simulink library "mpc555toucan"  (Simulink 6.0)
settings: Solver=ode45  SolverMode=SingleTasking  StartTime=0.0  StopTime=10.0  RelTol=1e-3
libraries: passthrough x20, driver_interface_library x10, canblocks x3, mpc555toucan x3, canblocks_extras x2, mpc555extras x2, mpc555interrupts x1, simulink x1, config_library x1
settings Model: Creator=The MathWorks Inc.  LastModifiedBy=batserve  ExtModeAutoUpdateStatusClock=off  ProdHWDeviceType=Specified
settings OptimizationCC: BooleanDataType=off
settings DebuggingCC: CheckExecutionContextPreStartOutputMsg=on  CheckExecutionContextRuntimeOutputMsg=on  SolverPrmCheckMsg=none
settings HardwareCC: ProdHWDeviceType=Specified  TargetUnknown=on

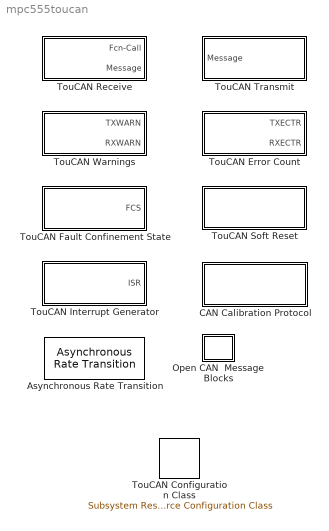
== system mpc555toucan ==
  Asynchronous Rate Transition : mpc555interrupts/Asynchronous Rate Transition  sample_time=-1
  CAN Calibration Protocol : Subsystem  TreatAsAtomicUnit=on  PropExecContextAcrossSSBoundary=on  mask(CAN Calibration Protocol (MPC555)){CCP_STATION_ID=hex2dec('1'), module=A, ccp_cro_id=hex2dec('6FA'), ccp_cro_message_type=Extended (29-bit identifier), ccp_return_id=hex2dec('6FB'), ccp_return_message_type=Extended (29-bit identifier), TOTAL_NUM_ODTS=8, cro_sample_time=0.01}
      mask prompts: CCP_STATION_ID "CCP station address (16-bit integer):"; module "TouCAN module:"; ccp_cro_id "CAN message identifier (CRO):"; ccp_cro_message_type "CAN message type (CRO):"; ccp_return_id "CAN message identifier (DTO/DAQ):"; ccp_return_message_type "CAN message type (DTO/DAQ):"; TOTAL_NUM_ODTS "Total Number of Object Descriptor Tables (ODTs):"; cro_sample_time "CRO sample time:"
      mask help:
      | Implements CAN Calibration Protocol (CCP v2.1) on the target processor.
      |
      | This block processes Command Receive Object (CRO) messages and outputs the resulting Data Transmission Object (DTO) and Data Acquisition (DAQ) messages.
      mask init:
      | % Propagate DAQ / DTO message type to underlying blocks
      | set_param([gcb, '/DAQ Processing/Send DAQ Message/CAN Message Packing'], 'message_type', ccp_return_message_type);
      | set_param([gcb, '/DTO Processing/CCP (Termination)/CAN Transmit/DTO_Constructor'], 'message_type', ccp_return_message_type);
      | % Propagate CRO message type to underlying blocks
      | set_param([gcb, '/TouCAN Receive'], 'message_type', ccp_cro_message_type);
      | % Propagate TouCAN module to underlying blocks
      | set_param([gcb, '/DAQ Processing/Send DAQ Message/TouCAN Transmit'], 'module', module);
      | set_param([gcb, '/DTO Processing/CCP (Termination)/CAN Transmit/TouCAN Transmit'], 'module', module);
      | set_param([gcb, '/TouCAN Receive'], 'module', module);
      | 
      | % check for a Resource Config block, and make sure it is MPC555
      | target = RTWConfigurationCB('get_target', gcb);
      | target.checkName('MPC555');
      | 
      | ccp_mpc555_init_mask('check_prog_prep_bit_timing', gcb, target);
      settings: CopyFcn=ccp_init_mask('copyfcn', gcb)
      mask Help: helpview([docroot '/toolbox/mpc555dk/mpc555dk.map'], 'target_CCP');
      mask StyleString: edit,popup(A|B|C),edit,popup(Standard (11-bit identifier)|Extended (29-bit identifier)),edit,popup(Standard (11-bit identifier)|Extended (29-bit identifier)),edit,edit
      mask Display: disp('CCP');
  Open CAN  Message Blocks : Subsystem  PropExecContextAcrossSSBoundary=on
      mask init:
      | [x colormap] = imread([matlabroot '\toolbox\rtw\targets\common\tgtcommon\model.gif']);
      | rgb = ind2rgb(x, colormap);
      settings: OpenFcn=canblocks
      mask Display: image(rgb)
  TouCAN Configuration Class : config_library/Subsystem Resource Configuration Class  Tag=CONFIGURATION DATA CLASS  dClassName=MPC555dkConfig.TOUCAN  rClassName=MPC555dkConfig.TOUCAN_RESOURCES
  TouCAN Error Count : Subsystem  PropExecContextAcrossSSBoundary=on  mask(MPC555 TouCAN Error Count (Transmit/Receive)){module=A, t=0.1, enablePassThru=off}
      mask prompts: t "Sample time:"; enablePassThru "Enable pass through (show simulation input)"
      mask help: Read the transmit/receive error counter registers (TXECTR/RXECTR) on the selected TouCAN module.
      mask init:
      | simulinkPortControl(gcbh,'enable','PassThroughRXECTR',enablePassThru);
      | simulinkPortControl(gcbh,'enable','PassThroughTXECTR',enablePassThru);
      | 
      | dispstr = sprintf('TouCAN_%s\nError Count', module);
      | 
      | if (enablePassThru)
      | 	passThroughDeprecationWarning;
      | end;
      | 
      | % check for a Resource Config block, and make sure it is MPC555
      | target = RTWConfigurationCB('get_target', gcb);
      | target.checkName('MPC555');
      | 
      | % Verify the modules selection is correct
      | mpc5xx_2can_verify_modules(gcb);
      mask Help: helpview([docroot '/toolbox/mpc555dk/mpc555dk.map'], 'TouCAN_Err_Ctr');
      mask StyleString: popup(A|B|C),edit,checkbox
      mask Display:
      | disp(dispstr)
      | port_label('output',1,'Tx');
      | port_label('output',2,'Rx');
  TouCAN Fault Confinement State : Subsystem  PropExecContextAcrossSSBoundary=on  mask(MPC555 TouCAN Fault Confinement State){module=A, t=0.1, enablePassThru=off}
      mask prompts: t "Sample time:"; enablePassThru "Enable pass through (show simulation input)"
      mask help: Indicates the fault confinement state of a TouCAN module.
      mask init:
      | simulinkPortControl(gcbh,'enable','PassThrough',enablePassThru);
      | 
      | dispstr = sprintf('TouCAN_%s\nFault \nConfinement State', module);
      | 
      | if (enablePassThru)
      | 	passThroughDeprecationWarning;
      | end;
      | 
      | % check for a Resource Config block, and make sure it is MPC555
      | target = RTWConfigurationCB('get_target', gcb);
      | target.checkName('MPC555');
      | 
      | % Verify the modules selection is correct
      | mpc5xx_2can_verify_modules(gcb);
      mask Help: helpview([docroot '/toolbox/mpc555dk/mpc555dk.map'], 'TouCAN_Fault');
      mask StyleString: popup(A|B|C),edit,checkbox
      mask Display: disp(dispstr)
  TouCAN Interrupt Generator : Subsystem  TreatAsAtomicUnit=on  PropExecContextAcrossSSBoundary=on  mask(MPC555 TouCAN Interrupt Generator){module=A, callback=Buffer 0, float_flag=on}
      mask prompts: callback "Interrupt source:"; float_flag "Use floating point"
      mask help:
      | Generate a function-call trigger within a TouCAN interrupt and execute a callback in the context of the interrupt service routine.
      |
      | Do not use this block in conjunction with the buffer that is used to transmit data as an interrupt is already generated for this buffer. If the callback does not contain floating-point data types, you can disable floating-point support for faster execution.
      mask init:
      | % check for a valid target block
      | driverBlock = regexprep(gcb, sprintf('\n'), ' ');
      | target = RTWConfigurationCB('get_target', driverBlock);
      | 
      | %Identifiy the callback ENUM used in the generated code
      | cbTypeHandle = findtype('MPC5XX_CAN_IRQ_SRCS');
      | cbTypes = cbTypeHandle.Strings;
      | callback_id = cbTypes{callback};
      | 
      | % Verify the modules selection is correct
      | mpc5xx_2can_verify_modules(gcb);
      | 
      | 
      | % Perform Resource Configuration
      | RTWConfiguration.Target.acquireResourceForBlock(      ...
      |    gcb,                    ...   % Current block
      |    'MPC555dkConfig.TOUCAN', ...   % Configuration Class
      |    ['CAN_' module '_IRQS'],          ...   % Resource Type associated with the configuration class
      |    callback_id,                    ...   % Resource being requested
      |    'TOUCAN Interrupt'            ...   % Lable to be used in error messages
      | );
      mask Help: helpview([docroot '/toolbox/mpc555dk/mpc555dk.map'], 'CAN_Interrupts');
      mask StyleString: popup(A|B|C),popup(Wake|Error|Bus off|Buffer 0|Buffer 1|Buffer 2|Buffer 3|Buffer 4|Buffer 5|Buffer 6|Buffer 7|Buffer 8|Buffer 9|Buffer 10|Buffer 11|Buffer 12|Buffer 13|Buffer 14|Buffer 15),checkbox
      mask Display: disp(sprintf('TouCAN_%s\nIRQ - %s', get_param(gcb,'module'), get_param(gcb,'callback')))
  TouCAN Receive : Subsystem  PropExecContextAcrossSSBoundary=on  mask(MPC555 TouCAN Receive){module=A, ids=hex2dec('0001'), notification_type=Function Call Outport, auto_select_buffer=on, bufferids=3, use_queue=off, queue_length=3, message_type=Standard (11-bit identifier), t=0.1}
      mask prompts: module "TouCAN module:"; ids "CAN message identifier:"; notification_type "New message notification via:"; auto_select_buffer "Automatically select buffer"; bufferids "Buffer number [0 -15]:"; use_queue "Use interrupt driven queue to buffer received messages"; queue_length "Length (number of messages) of interrupt driven queue:"; message_type "CAN message type:"; t "Sample time:"
      mask help: Receives CAN messages from the selected TouCAN module.
      mask init:
      | % Show the trigger port
      | show_trigger = notification_type == 1 ;
      | 
      | % enable / disable ports
      | simulinkPortControl(gcbh,'enable','FcnCallOutput',show_trigger);
      | 
      | dispstr = sprintf('TouCAN_%s\nReceive',get_param(gcb,'module'));
      | 
      | % check for a Resource Config block, and make sure it is MPC555
      | target = RTWConfigurationCB('get_target', gcb);
      | target.checkName('MPC555');
      | 
      | % Verify the modules selection is correct
      | mpc5xx_2can_verify_modules(gcb);
      | 
      | % Possibly auto-allocate the buffer
      | bufferids = mask_resource_validator(gcb,@mpc555_canrx_validate, bufferids);
      | 
      | % check for valid CAN message identifier
      | can_msg_id_check(ids,message_type);
      | message_type=message_type-1;
      | module=module-1;
      | 
      | % check queue params
      | if use_queue==1
      | 	if (length(queue_length)~= 1) | (queue_length <= 0) | (floor(queue_length)~=queue_length)
      | 		error('The queue length parameter must an integer greater than zero');
      | 	end
      | end
      | 
      | % Setup the mask display
      | if show_trigger
      | 	md = sprintf('disp(dispstr);\nport_label(''output'',1,''f()'');\nport_label(''output'',2,''Msg'');');
      | else
      | 	md = sprintf('disp(dispstr);\nport_label(''output'',1,''Msg'');');
      | end
      | set_param(gcb,'MaskDisplay',md);
      | 
      | if use_queue
      | 	% Perform Resource Configuration
      | 	resource_type = sprintf('CAN_%s_IRQS', get_param(gcb,'module'));
      | 	resource = sprintf('CAN_IRQ_BUFFER%d',bufferids);
      | 	RTWConfiguration.Target.aquireResourceForBlock(      ...
      |    		gcb,                    ...   % Current block
      |    		'MPC555dkConfig.TOUCAN', ...   % Configuration Class
      |    		resource_type,          ...   % Resource Type associated with the configuration class
      |    		resource,                    ...   % Resource being requested
      |    		'CAN Interrupt'            ...   % Lable to be used in error messages
      | 	);
      | end
      mask Help: helpview([docroot '/toolbox/mpc555dk/mpc555dk.map'], 'TouCAN_RX');
      mask StyleString: popup(A|B|C),edit,popup(Function Call Outport|'TouCAN Interrupt Generator' Block),checkbox,edit,checkbox,edit,popup(Standard (11-bit identifier)|Extended (29-bit identifier)),edit
      mask CallbackString:
      | ||tempFcnIrq = get_param(gcb,'notification_type');
      | switch tempFcnIrq
      | 	case 'Function Call Outport'
      | 	    simUtil_maskParam('enable',gcb,'use_queue');
      | 		simUtil_maskParam('enable',gcb,'auto_select_buffer');
      | 	otherwise
      | 	    simUtil_maskParam('disable',gcb,'use_queue');
      | 		simUtil_maskParam('disable',gcb,'queue_length');
      |         set_param(gcb,'use_queue','off');
      | 
      | 		set_param(gcb,'auto_select_buffer','off');
      | 		simUtil_maskParam('disable',gcb,'auto_select_buffer');
      | 		simUtil_maskParam('enable',gcb,'bufferids');
      | end
      | clear tempFcnIrq|tempCanRxASB = get_param(gcb,'auto_select_buffer');
      | switch tempCanRxASB
      | 	case 'on'
      | 		simUtil_maskParam('disable',gcb,'bufferids');
      | 	case 'off'
      | 	    simUtil_maskParam('enable',gcb,'bufferids');
      | end
      | clear tempCanRxASB||tempCanRxUseQ = get_param(gcb,'use_queue');
      | switch tempCanRxUseQ
      | 	case 'on'
      | 		simUtil_maskParam('enable',gcb,'queue_length');
      |     case 'off'
      | 	    simUtil_maskParam('disable',gcb,'queue_length');
      | end
      | clear tempCanRxUseQ|||
      mask Display:
      | disp(dispstr)
      | port_label('output',1,'f()');
      | port_label('output',2,'Msg');
  TouCAN Soft Reset : Subsystem  TreatAsAtomicUnit=on  PropExecContextAcrossSSBoundary=on  mask(MPC555 TouCAN Soft Reset){module=A, t=-1}
      mask prompts: t "Sample time:"
      mask help:
      | Performs a TouCAN module soft reset and re-initialization. All error counters and error flags are reset during this process, but the contents of the message buffers and the transmit queue are unchanged.
      |
      | This block should be placed in a triggered or function-call subsystem.
      mask init:
      | dispstr = sprintf('TouCAN_%s\nSoft Reset', module);
      | 
      | % check for a Resource Config block, and make sure it is MPC555
      | target = RTWConfigurationCB('get_target', gcb);
      | target.checkName('MPC555');
      | 
      | % Verify the modules selection is correct
      | mpc5xx_2can_verify_modules(gcb);
      mask Help: helpview([docroot '/toolbox/mpc555dk/mpc555dk.map'], 'TouCAN_Reset');
      mask StyleString: popup(A|B|C),edit
      mask Display: disp(dispstr)
  TouCAN Transmit : Subsystem  PropExecContextAcrossSSBoundary=on  mask(MPC555 TouCAN Transmit){module=A, tx_mode=Queued transmission with shared buffer, fifo_queue_length=8, bufferids=0, t=-1, enablePassThru=off}
      mask prompts: tx_mode "Transmit mode:"; fifo_queue_length "Length (number of messages) of FIFO queue:"; bufferids "Buffers (hidden)"; t "Sample time:"; enablePassThru "Enable pass through (show simulation output)"
      mask help: Transmits a CAN message via the selected TouCAN module.
      mask init:
      | simulinkPortControl(gcbh,'enable','PassThrough',enablePassThru);
      | 
      | dispstr=sprintf('TouCAN_%s\nTransmit', get_param(gcb,'module'));
      | 
      | if (enablePassThru)
      | 	passThroughDeprecationWarning;
      | end;
      | 
      | % check for a Resource Config block, and make sure it is MPC555
      | target = RTWConfigurationCB('get_target', gcb);
      | target.checkName('MPC555');
      | 
      | % verify the modules selection is correct
      | mpc5xx_2can_verify_modules(gcb);
      | 
      | % Possibly autoallocate the buffer
      | bufferids = mask_resource_validator(gcb,@mpc555_cantx_validate,bufferids);
      | 
      | module=module-1;
      mask Help: helpview([docroot '/toolbox/mpc555dk/mpc555dk.map'], 'TouCAN_TX');
      mask StyleString: popup(A|B|C),popup(Queued transmission with shared buffer|Direct transmission with dedicated buffer|FIFO queued transmission with dedicated buffer),edit,edit,edit,checkbox
      mask CallbackString:
      | |tempCanTxTxMode = get_param(gcb,'tx_mode');
      | switch tempCanTxTxMode
      | 	case {'Queued transmission with shared buffer','Direct transmission with dedicated buffer'}
      | 		simUtil_maskParam('hide',gcb,'fifo_queue_length');
      |     case 'FIFO queued transmission with dedicated buffer'
      | 	    simUtil_maskParam('show',gcb,'fifo_queue_length');
      | 	otherwise
      | 		error(['Unrecognized value for tx_mode in ' gcb ]);
      | end
      | clear tempCanTxTxMode||||
      mask Display:
      | disp(dispstr)
      | port_label('input',1,'Msg');
  TouCAN Warnings : Subsystem  PropExecContextAcrossSSBoundary=on  mask(MPC555 TouCAN Warnings (Transmit/Receive)){module=A, t=0.1, enablePassThru=off}
      mask prompts: t "Sample time:"; enablePassThru "Enable pass through (show simulation input)"
      mask help:
      | Read the transmit/receive warning bits (TXWARN/RXWARN) from the error and status register (ESTAT) on the selected TouCAN module.
      |
      | If the transmit/receive error counter exceeds 95 then the TXWARN/RXWARN output goes high.
      mask init:
      | simulinkPortControl(gcbh,'enable','PassThroughRX',enablePassThru);
      | simulinkPortControl(gcbh,'enable','PassThroughTX',enablePassThru);
      | 
      | dispstr = sprintf('TouCAN_%s\nWarnings', module);
      | 
      | if (enablePassThru)
      | 	passThroughDeprecationWarning;
      | end;
      | 
      | % check for a Resource Config block, and make sure it is MPC555
      | target = RTWConfigurationCB('get_target', gcb);
      | target.checkName('MPC555');
      | 
      | % Verify the modules selection is correct
      | mpc5xx_2can_verify_modules(gcb);
      mask Help: helpview([docroot '/toolbox/mpc555dk/mpc555dk.map'], 'TouCAN_Warn');
      mask StyleString: popup(A|B|C),edit,checkbox
      mask Display:
      | disp(dispstr)
      | port_label('output',1,'Tx');
      | port_label('output',2,'Rx');

== system mpc555toucan/CAN Calibration Protocol ==
  DAQ Processing : Subsystem  PropExecContextAcrossSSBoundary=on
      mask Display: disp('DAQ');
  DTO Processing : Subsystem  TreatAsAtomicUnit=on  PropExecContextAcrossSSBoundary=on
      mask Display: disp('DTO');
  TouCAN Receive : mpc555toucan/TouCAN Receive  module=A  ids=ccp_cro_id  notification_type=Function Call Outport  auto_select_buffer=on  bufferids=14  use_queue=off  queue_length=3  message_type=Extended (29-bit identifier)  t=cro_sample_time
  wires:
  TouCAN Receive/1 -> DTO Processing/Trigger
  TouCAN Receive/2 -> DTO Processing/1(CRO)

== system mpc555toucan/Open CAN  Message Blocks ==

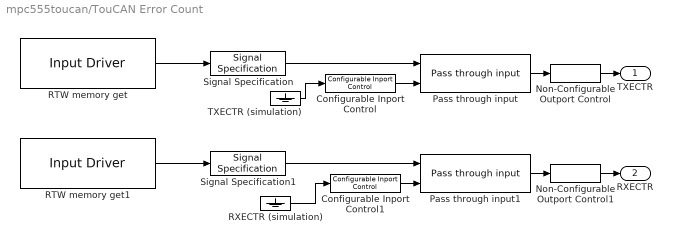
== system mpc555toucan/TouCAN Error Count ==
  Configurable Inport Control : passthrough/Configurable Inport Control  portNum=1  portName=PassThroughTXECTR  isEnabled=0  isConfigurable=1  isInport=1
  Configurable Inport Control1 : passthrough/Configurable Inport Control  portNum=2  portName=PassThroughRXECTR  isEnabled=0  isConfigurable=1  isInport=1
  Non-Configurable Outport Control : passthrough/Non-Configurable Outport Control  portNum=1  isEnabled=1  isConfigurable=0  isInport=0
  Non-Configurable Outport Control1 : passthrough/Non-Configurable Outport Control  portNum=2  isEnabled=1  isConfigurable=0  isInport=0
  Pass through input : passthrough/Pass through input
  Pass through input1 : passthrough/Pass through input
  RTW memory get : driver_interface_library/Input Driver  t=t  expr=['CAN_', module, '.TXECTR.R']  portWidth=1  pOpt=[]  expression_type=Expression
  RTW memory get1 : driver_interface_library/Input Driver  t=t  expr=['CAN_', module, '.RXECTR.R']  portWidth=1  pOpt=[]  expression_type=Expression
  RXECTR (simulation) : Ground
  Signal Specification : SignalSpecification  DataType=uint8
  Signal Specification1 : SignalSpecification  DataType=uint8
  TXECTR (simulation) : Ground
  TXECTR : Outport
  RXECTR : Outport  Port=2
  wires:
  Non-Configurable Outport Control1/1 -> RXECTR/1
  Non-Configurable Outport Control/1 -> TXECTR/1
  Configurable Inport Control1/1 -> Pass through input1/2
  Configurable Inport Control/1 -> Pass through input/2
  RTW memory get/1 -> Signal Specification/1
  RTW memory get1/1 -> Signal Specification1/1
  Pass through input1/1 -> Non-Configurable Outport Control1/1
  RXECTR (simulation)/1 -> Configurable Inport Control1/1
  Pass through input/1 -> Non-Configurable Outport Control/1
  TXECTR (simulation)/1 -> Configurable Inport Control/1
  Signal Specification1/1 -> Pass through input1/1
  Signal Specification/1 -> Pass through input/1

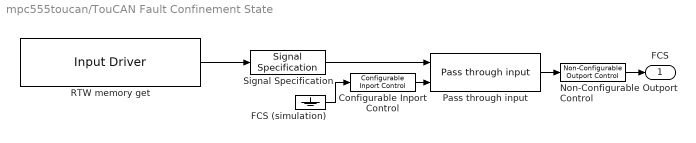
== system mpc555toucan/TouCAN Fault Confinement State ==
  Configurable Inport Control : passthrough/Configurable Inport Control  portNum=1  portName=PassThrough  isEnabled=0  isConfigurable=1  isInport=1
  FCS (simulation) : Ground
  Non-Configurable Outport Control : passthrough/Non-Configurable Outport Control  portNum=1  isEnabled=1  isConfigurable=0  isInport=0
  Pass through input : passthrough/Pass through input
  RTW memory get : driver_interface_library/Input Driver  t=t  expr=['CAN_', module, '.ESTAT.B.FCS']  portWidth=1  pOpt=[]  expression_type=Expression
  Signal Specification : SignalSpecification  Dimensions=1  DataType=uint16
  FCS : Outport
  wires:
  Non-Configurable Outport Control/1 -> FCS/1
  Configurable Inport Control/1 -> Pass through input/2
  RTW memory get/1 -> Signal Specification/1
  Pass through input/1 -> Non-Configurable Outport Control/1
  FCS (simulation)/1 -> Configurable Inport Control/1
  Signal Specification/1 -> Pass through input/1

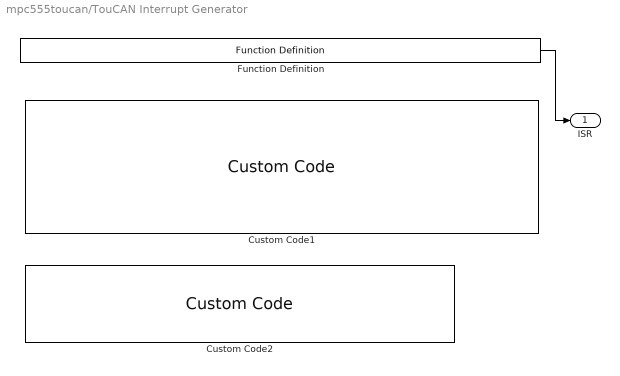
== system mpc555toucan/TouCAN Interrupt Generator ==
  Custom Code1 : driver_interface_library/Custom Code
  Custom Code2 : driver_interface_library/Custom Code
  Function Definition : driver_interface_library/Function Definition  function_name=[ 'void can_irq_CAN_' module '_' callback_id '(PCAN_MODULE module, TOUCAN_IRQ_SOURCE source )']
  ISR : Outport
  wires:
  Function Definition/1 -> ISR/1

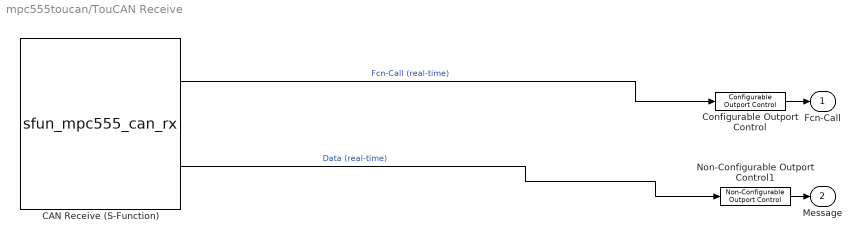
== system mpc555toucan/TouCAN Receive ==
  CAN Receive (S-Function) : S-Function  FunctionName=sfun_mpc555_can_rx  Parameters=module uint32(ids) t message_type uint32(bufferids) use_queue queue_length notification_type
  Configurable Outport Control : passthrough/Configurable Outport Control  portNum=1  portName=FcnCallOutput  isEnabled=1  isConfigurable=1  isInport=0
  Non-Configurable Outport Control1 : passthrough/Non-Configurable Outport Control  portNum=2  isEnabled=1  isConfigurable=0  isInport=0
  Fcn-Call : Outport
  Message : Outport  Port=2
  wires:
  CAN Receive (S-Function)/2 -> Non-Configurable Outport Control1/1  "Data (real-time)"
  CAN Receive (S-Function)/1 -> Configurable Outport Control/1  "Fcn-Call (real-time)"
  Configurable Outport Control/1 -> Fcn-Call/1
  Non-Configurable Outport Control1/1 -> Message/1

== system mpc555toucan/TouCAN Soft Reset ==
  Extended Custom Code : mpc555extras/Extended Custom Code
  Extended Custom Code1 : mpc555extras/Extended Custom Code

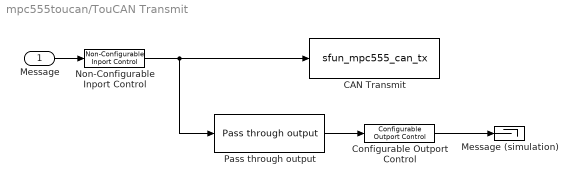
== system mpc555toucan/TouCAN Transmit ==
  Message : Inport  Port=1  LatchInput=off
  CAN Transmit : S-Function  FunctionName=sfun_mpc555_can_tx  Parameters=module, t, tx_mode, uint32(bufferids), fifo_queue_length
  Configurable Outport Control : passthrough/Configurable Outport Control  portNum=1  portName=PassThrough  isEnabled=0  isConfigurable=1  isInport=0
  Message (simulation) : Terminator
  Non-Configurable Inport Control : passthrough/Non-Configurable Inport Control  portNum=1  isEnabled=1  isConfigurable=0  isInport=1
  Pass through output : passthrough/Pass through output  driverBlock=gcs
  wires:
  Message/1 -> Non-Configurable Inport Control/1
  Pass through output/1 -> Configurable Outport Control/1
  Configurable Outport Control/1 -> Message (simulation)/1
  Non-Configurable Inport Control/1 -> CAN Transmit/1, Pass through output/1

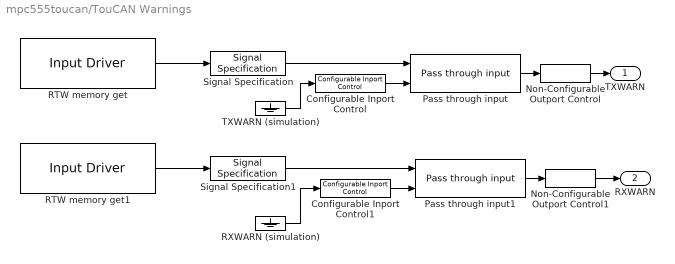
== system mpc555toucan/TouCAN Warnings ==
  Configurable Inport Control : passthrough/Configurable Inport Control  portNum=1  portName=PassThroughTX  isEnabled=0  isConfigurable=1  isInport=1
  Configurable Inport Control1 : passthrough/Configurable Inport Control  portNum=2  portName=PassThroughRX  isEnabled=0  isConfigurable=1  isInport=1
  Non-Configurable Outport Control : passthrough/Non-Configurable Outport Control  portNum=1  isEnabled=1  isConfigurable=0  isInport=0
  Non-Configurable Outport Control1 : passthrough/Non-Configurable Outport Control  portNum=2  isEnabled=1  isConfigurable=0  isInport=0
  Pass through input : passthrough/Pass through input
  Pass through input1 : passthrough/Pass through input
  RTW memory get : driver_interface_library/Input Driver  t=t  expr=['CAN_', module, '.ESTAT.B.TXWARN']  portWidth=1  pOpt=[]  expression_type=Expression
  RTW memory get1 : driver_interface_library/Input Driver  t=t  expr=['CAN_', module, '.ESTAT.B.RXWARN']  portWidth=1  pOpt=[]  expression_type=Expression
  RXWARN (simulation) : Ground
  Signal Specification : SignalSpecification  DataType=boolean
  Signal Specification1 : SignalSpecification  DataType=boolean
  TXWARN (simulation) : Ground
  TXWARN : Outport
  RXWARN : Outport  Port=2
  wires:
  Non-Configurable Outport Control1/1 -> RXWARN/1
  Non-Configurable Outport Control/1 -> TXWARN/1
  Configurable Inport Control1/1 -> Pass through input1/2
  Configurable Inport Control/1 -> Pass through input/2
  Pass through input/1 -> Non-Configurable Outport Control/1
  RTW memory get1/1 -> Signal Specification1/1
  RTW memory get/1 -> Signal Specification/1
  Pass through input1/1 -> Non-Configurable Outport Control1/1
  RXWARN (simulation)/1 -> Configurable Inport Control1/1
  Signal Specification1/1 -> Pass through input1/1
  TXWARN (simulation)/1 -> Configurable Inport Control/1
  Signal Specification/1 -> Pass through input/1

== system mpc555toucan/CAN Calibration Protocol/DAQ Processing ==
  note: Must use "RTW memory get" block to access the msg_pointer
  Function Definition : driver_interface_library/Function Definition  function_name='void exported_ccp_daq_trigger(uint8_T * msg_pointer)'
  Send DAQ Message : Subsystem  TreatAsAtomicUnit=on  PropExecContextAcrossSSBoundary=on
      mask Type: Send DAQ Message
  wires:
  Function Definition/1 -> Send DAQ Message/Trigger

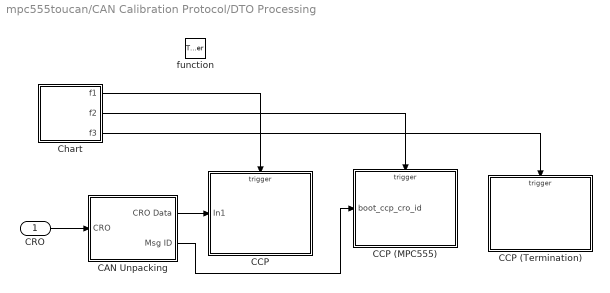
== system mpc555toucan/CAN Calibration Protocol/DTO Processing ==
  CRO : Inport  Port=1  LatchInput=off
  function : TriggerPort  TriggerType=function-call
  CAN Unpacking : Subsystem  PropExecContextAcrossSSBoundary=on
  CCP : Subsystem  TreatAsAtomicUnit=on  PropExecContextAcrossSSBoundary=on
      mask Type: CCP
  CCP (MPC555) : Subsystem  TreatAsAtomicUnit=on  PropExecContextAcrossSSBoundary=on
  CCP (Termination) : Subsystem  TreatAsAtomicUnit=on  PropExecContextAcrossSSBoundary=on
      mask Type: CCP (Termination)
  Chart : Stateflow chart  PropExecContextAcrossSSBoundary=on
  wires:
  CAN Unpacking/2(Msg ID) -> CCP (MPC555)/1(boot_ccp_cro_id)
  CAN Unpacking/1(CRO Data) -> CCP/1(In1)
  CRO/1 -> CAN Unpacking/1(CRO)
  Chart/1(f1) -> CCP/Trigger
  Chart/2(f2) -> CCP (MPC555)/Trigger
  Chart/3(f3) -> CCP (Termination)/Trigger

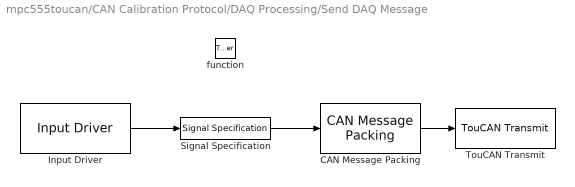
== system mpc555toucan/CAN Calibration Protocol/DAQ Processing/Send DAQ Message ==
  function : TriggerPort  TriggerType=function-call
  CAN Message Packing : canblocks/CAN Message Packing  id=ccp_return_id  message_type=Extended (29-bit identifier)  endian=Little Endian (Intel)
  Input Driver : driver_interface_library/Input Driver  t=-1  expr='msg_pointer[%<i>]'  portWidth=8  pOpt=[]  expression_type=Not expression
  Signal Specification : SignalSpecification  DataType=uint8
  TouCAN Transmit : mpc555toucan/TouCAN Transmit  module=A  tx_mode=FIFO queued transmission with dedicated buffer  fifo_queue_length=8  bufferids=0  t=-1  enablePassThru=off
  wires:
  Input Driver/1 -> Signal Specification/1
  Signal Specification/1 -> CAN Message Packing/1
  CAN Message Packing/1 -> TouCAN Transmit/1

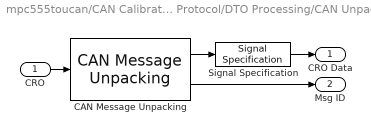
== system mpc555toucan/CAN Calibration Protocol/DTO Processing/CAN Unpacking ==
  CRO : Inport  Port=1  LatchInput=off
  CAN Message Unpacking : canblocks/CAN Message Unpacking/CAN Message Unpacking  showData=on  showID=on  showLength=off  endian=Little Endian (Intel)
  Signal Specification : simulink/Signal Attributes/Signal Specification  D=8  Ts=-1  DataType=uint8  OutDataType=sfix(16)  OutScaling=2^0
      settings: SignalType=auto  SamplingMode=auto
  CRO Data : Outport
  Msg ID : Outport  Port=2
  wires:
  CAN Message Unpacking/2 -> Msg ID/1
  CAN Message Unpacking/1 -> Signal Specification/1
  CRO/1 -> CAN Message Unpacking/1
  Signal Specification/1 -> CRO Data/1

== system mpc555toucan/CAN Calibration Protocol/DTO Processing/CCP ==
  In1 : Inport  Port=1  LatchInput=off
  function : TriggerPort  TriggerType=function-call
  CAN Calibration Protocol : canblocks_extras/CAN Calibration Protocol  CCP_STATION_ID=CCP_STATION_ID  TOTAL_NUM_ODTS=TOTAL_NUM_ODTS  show_commands=off  GET_CCP_VERSIONenabled=on  EXCHANGE_IDenabled=on  SET_MTAenabled=on  DNLOADenabled=on  DNLOAD_6enabled=on  UPLOADenabled=on  SHORT_UPenabled=on  GET_DAQ_SIZEenabled=on  SET_DAQ_PTRenabled=on  WRITE_DAQenabled=on  START_STOPenabled=on  SET_S_STATUSenabled=on  GET_S_STATUSenabled=on  START_STOP_ALLenabled=on
      settings: AttributesFormatString=\n\n
  wires:
  In1/1 -> CAN Calibration Protocol/1

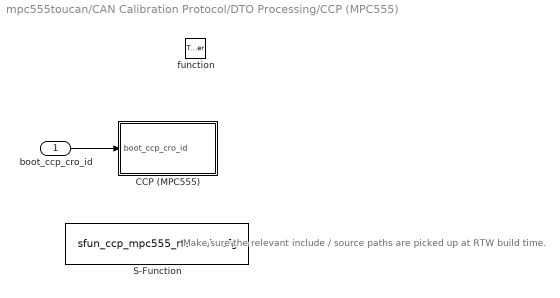
== system mpc555toucan/CAN Calibration Protocol/DTO Processing/CCP (MPC555) ==
  note: Make sure the relevant
      | include / source paths are picked up
      | at RTW build time.
  boot_ccp_cro_id : Inport  Port=1  LatchInput=off
  function : TriggerPort  TriggerType=function-call
  CCP (MPC555) : Subsystem  PropExecContextAcrossSSBoundary=on  mask{boot_ccp_dto_id=ccp_return_id, show_commands=off, PROGRAM_PREPAREenabled=on, DNLOADenabled=off, DNLOAD_6enabled=off, UPLOADenabled=off, SHORT_UPenabled=off}
      mask prompts: show_commands "Enable / Disable Connected State Commands"; PROGRAM_PREPAREenabled "PROGRAM_PREPARE"; DNLOADenabled "DNLOAD (with MPC555 Interrupt Disable / Enable)"; DNLOAD_6enabled "DNLOAD_6 (with MPC555 Interrupt Disable / Enable)"; UPLOADenabled "UPLOAD (with MPC555 Interrupt Disable / Enable)"; SHORT_UPenabled "SHORT_UP (with MPC555 Interrupt Disable / Enable)"
      mask CallbackString: |ccp_mpc555_init_mask('show_commands_mask_callback',gcbh);|||||
  S-Function : S-Function  FunctionName=sfun_ccp_mpc555_rtwmakecfg
  wires:
  boot_ccp_cro_id/1 -> CCP (MPC555)/1(boot_ccp_cro_id)

== system mpc555toucan/CAN Calibration Protocol/DTO Processing/CCP (Termination) ==
  function : TriggerPort  TriggerType=function-call
  CAN Calibration Protocol (Termination) : canblocks_extras/CAN Calibration Protocol (Termination)
      settings: AttributesFormatString=\n\n
  CAN Transmit : Subsystem  TreatAsAtomicUnit=on  PropExecContextAcrossSSBoundary=on
      mask Type: CAN Transmit
  wires:
  CAN Calibration Protocol (Termination)/2 -> CAN Transmit/1(DTO Data)
  CAN Calibration Protocol (Termination)/1 -> CAN Transmit/Trigger

== system mpc555toucan/CAN Calibration Protocol/DTO Processing/CCP (MPC555)/CCP (MPC555) ==
  boot_ccp_cro_id : Inport  Port=1  LatchInput=off
  CCP_MPC555 : Stateflow chart  PropExecContextAcrossSSBoundary=on
  wires:
  boot_ccp_cro_id/1 -> CCP_MPC555/1(boot_ccp_cro_id)

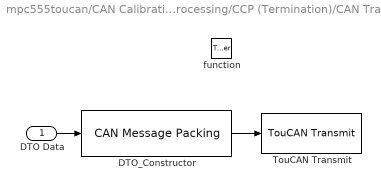
== system mpc555toucan/CAN Calibration Protocol/DTO Processing/CCP (Termination)/CAN Transmit ==
  DTO Data : Inport  Port=1  LatchInput=off
  function : TriggerPort  TriggerType=function-call
  DTO_Constructor : canblocks/CAN Message Packing  id=ccp_return_id  message_type=Extended (29-bit identifier)  endian=Little Endian (Intel)
  TouCAN Transmit : mpc555toucan/TouCAN Transmit  module=A  tx_mode=Queued transmission with shared buffer  fifo_queue_length=8  bufferids=0  t=-1  enablePassThru=off
  wires:
  DTO Data/1 -> DTO_Constructor/1
  DTO_Constructor/1 -> TouCAN Transmit/1

== stateflow chart CAN Calibration Protocol/DTO Processing/CCP (MPC555)/CCP (MPC555)/CCP_MPC555 ==
  note: Force target to start executing boot code, ready for a CAN download
  note: Read up to 5 bytes from memory.
  note: Write up to 5 bytes to memory.
  state tx_dto(tx_comm_type) [function]
    note: Flag to other blocks that this block could deal with the command.
    note: Returns data read from the target. Using MTA.
    note: Returns data read from the target. From specified address.
    note: Returns the current mta -
        | using get_mta()
    (default) -> (junction 26) : {setHandled(1);}
    (junction 26) -> (junction 24) : [(tx_comm_type==CCP_DNLOAD) || (tx_comm_type==CCP_DNLOAD_6)]
        | {c_getUINT32bytes(getMTAPtr(0),getDataPtr(4));
        | setData(3,MTA_ADDRESS_EXTENSION);
        | setData(2,getData(1));
        | setData(1,CCP_CRC_OK);
        | setData(0,CCP_DTO_ID);}
    (junction 26) -> (junction 23)
    (junction 23) -> (junction 25) : [tx_comm_type==CCP_SHORT_UPLOAD]
        | {c_setUINT32bytes(&memptr, getDataPtr(4));
        | EID();
        | c_read_uint8s(getDataPtr(3),getData(2), &memptr);
        | EIE();
        | setData(2,getData(1));
        | setData(1,CCP_CRC_OK);
        | setData(0,CCP_DTO_ID);
        | }
    (junction 28) -> (junction 27) : [tx_comm_type==CCP_UPLOAD]
        | {EID();
        | c_read_uint8s(getDataPtr(3),getData(2),getMTAPtr(0));
        | EIE();
        | setData(2,getData(1));
        | setData(1,CCP_CRC_OK);
        | setData(0,CCP_DTO_ID);}
    (junction 23) -> (junction 28)
  (default) -> (junction 11) : [(getHandled()==0) && (getCurrent_State()==CCP_CONNECTED_STATE)]
  (junction 11) -> (junction 12)
  (junction 12) -> (junction 13) : [PROGRAM_PREPAREenabled && (getData(0)==CCP_PROGRAM_PREPARE)]
      | {setHandled(1);
      | c_program_prepare(boot_ccp_cro_id, boot_ccp_dto_id, getData(0), getData(1), getData(2), getData(3), getData(4), getData(5), getData(6), getData(7));}
  (junction 16) -> (junction 14) : {setHandled(0);}
  (junction 16) -> (junction 15) : [UPLOADenabled && (getData(0)==CCP_UPLOAD)]
      | {tx_dto(CCP_UPLOAD);}
  (junction 17) -> (junction 16)
  (junction 19) -> (junction 17)
  (junction 21) -> (junction 19)
  (junction 12) -> (junction 21)
  (junction 19) -> (junction 18) : [DNLOAD_6enabled && (getData(0)==CCP_DNLOAD_6)]
      | {EID();
      | c_write_uint8s(getDataPtr(2),6,getMTAPtr(0));
      | EIE();
      | tx_dto(CCP_DNLOAD_6);}
  (junction 17) -> (junction 22) : [SHORT_UPenabled && (getData(0)==CCP_SHORT_UPLOAD)]
      | {tx_dto(CCP_SHORT_UPLOAD);}
  (junction 21) -> (junction 20) : [DNLOADenabled && (getData(0)==CCP_DNLOAD)]
      | {EID();
      | c_write_uint8s(getDataPtr(3),getData(2),getMTAPtr(0));
      | EIE();
      | tx_dto(CCP_DNLOAD);}
  data: memptr temporary uint32 size=1; tx_comm_type function_input double size=1; MTA_ADDRESS_EXTENSION constant uint8 size=1; boot_ccp_dto_id local uint32 size=1; PROGRAM_PREPAREenabled parameter boolean size=1; DNLOADenabled parameter boolean size=1; UPLOADenabled parameter boolean size=1; SHORT_UPenabled parameter boolean size=1; DNLOAD_6enabled parameter boolean size=1; boot_ccp_cro_id input uint32 size=1

== stateflow chart CAN Calibration Protocol/DTO Processing/Chart ==
  (default) -> (junction 59) : {f1;f2;f3;}
  events: f1 output FUNCTION_CALL_EVENT; f2 output FUNCTION_CALL_EVENT; f3 output FUNCTION_CALL_EVENT
